simulink model "Engine"  (R2023b)
settings: Solver=VariableStepAuto  StartTime=0.0  StopTime=10.0  RelTol=1e-3
undefined symbols (not defined in the file or in its folder): CT_ref, CT_table, Ma, Mach_bp, N1_bp, N1_idle, N1_lim, T_static
settings Model: Creator=24034  LastModifiedBy=24034

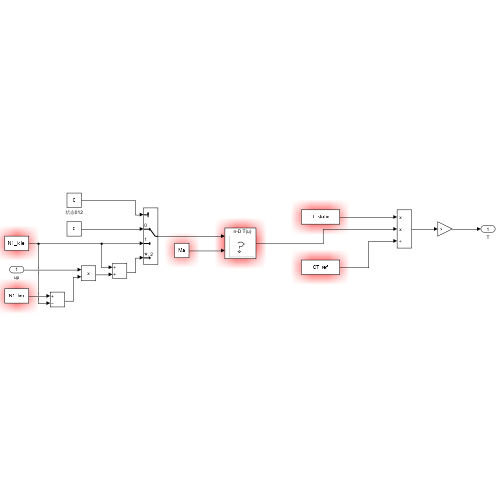
[thumbnail: Simulink's stored preview of the top-level diagram]
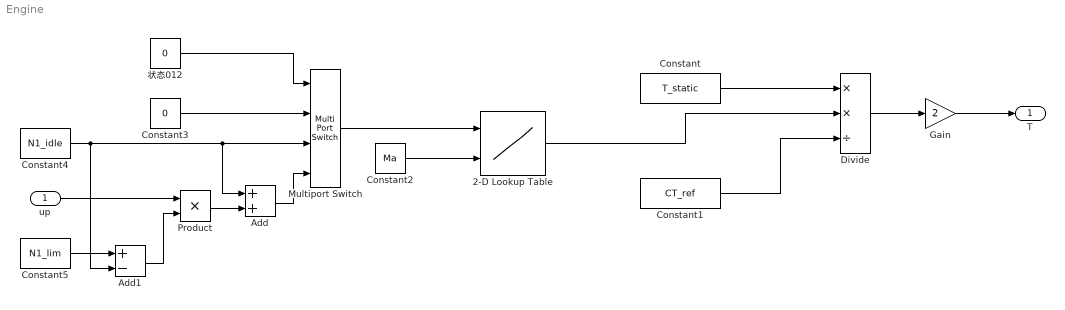
== system Engine ==
  up : Inport
  2-D Lookup Table : Lookup_n-D  BreakpointsForDimension1=N1_bp  BreakpointsForDimension2=Mach_bp  Table=CT_table  InternalRulePriority=Speed  RndMeth=Simplest
      settings: InputPortMap=u0,u1
  Add : Sum
  Add1 : Sum  Inputs=+-
  Constant : Constant  Value=T_static
  Constant1 : Constant  Value=CT_ref
  Constant2 : Constant  Value=Ma
  Constant3 : Constant  Value=0
  Constant4 : Constant  Value=N1_idle
  Constant5 : Constant  Value=N1_lim
  Divide : Product  Inputs=**/
  Gain : Gain  Gain=2
  Multiport Switch : MultiPortSwitch  DataPortOrder=Zero-based contiguous  zeroidx=on  SaturateOnIntegerOverflow=off  InputSameDT=off
  Product : Product
  状态012 : Constant  Value=0
  T : Outport
  wires:
  Constant/1 -> Divide/1
  Constant1/1 -> Divide/3
  Multiport Switch/1 -> 2-D Lookup Table/1
  Constant2/1 -> 2-D Lookup Table/2
  2-D Lookup Table/1 -> Divide/2
  Divide/1 -> Gain/1
  Gain/1 -> T/1
  状态012/1 -> Multiport Switch/1
  Constant4/1 -> Add1/2, Add/1, Multiport Switch/3
  Product/1 -> Add/2
  up/1 -> Product/1
  Add1/1 -> Product/2
  Constant5/1 -> Add1/1
  Constant3/1 -> Multiport Switch/2
  Add/1 -> Multiport Switch/4
